simulink model "testManyBound1"  (Simulink 7.4)
settings: Solver=ode45  StartTime=0.0  StopTime=10.0  RelTol=1e-3
libraries: BLOM_Lib x3
settings Model: Creator=Eric  LastModifiedBy=Eric

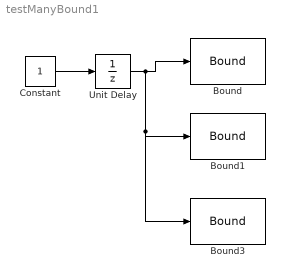
== system testManyBound1 ==
  Bound : BLOM_Lib/Bound  SystemSampleTime=-1  ub=1  lb=0  initial_step=off  final_step=off  intermediate_step=off
  Bound1 : BLOM_Lib/Bound  SystemSampleTime=-1  ub=2  lb=1  initial_step=off  final_step=off  intermediate_step=on
  Bound3 : BLOM_Lib/Bound  SystemSampleTime=-1  ub=3  lb=2  initial_step=off  final_step=on  intermediate_step=off
  Constant : Constant  OutDataType=fixdt(1, 16)  OutScaling=2^0
  Unit Delay : UnitDelay  SampleTime=-1
  wires:
  Constant/1 -> Unit Delay/1
  Unit Delay/1 -> Bound/1, Bound1/1, Bound3/1
